simulink model "ACC"  (Simulink 7.4)
settings: Solver=ode45  StartTime=0.0  StopTime=100  RelTol=1e-3
values from neighbouring files (symbols this model uses):
  A = ACC_cont.A    [pritam_acc.m]
  ACCController_name = 'ACCController'    [pritam_acc.m]
  B = ACC_cont.B    [pritam_acc.m]
  Bd = ACC_cont.C    [pritam_acc.m]
  uini = 0    [pritam_acc.m]
  xini = [40;29;30]    [pritam_acc.m]
libraries: simulink x1
settings Model: Creator=manuelmazo  LastModifiedBy=p261584  ExtModeAutoUpdateStatusClock=off
settings OptimizationCC: InitFltsAndDblsToZero=on
settings DebuggingCC: SaveWithParameterizedLinksMsg=none
settings GRTTargetCC: TargetFcnLib=ansi_tfl_tmw.mat

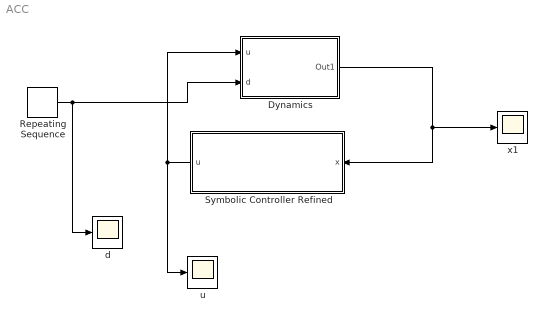
== system ACC ==
  Dynamics : Subsystem
  Repeating Sequence : simulink/Sources/Repeating Sequence  SystemSampleTime=-1  rep_seq_t=[0 0.2]  rep_seq_y=[-0.1 -0.1]
  Symbolic Controller Refined : Subsystem  mask{contr_name=ACCController_name, uini=uini}
      mask prompts: contr_name "Controller Name"; uini "Initial Controller State"
      mask init:
      | load(strcat(contr_name,'_symb'), 'params_symb');
  d : Scope
      settings: YMin=-0.1  YMax=-0.1
  u : Scope
      settings: YMin=-1  YMax=1  SaveName=ScopeData3
  x1 : Scope
      settings: YMin=25  YMax=65
  wires:
  Dynamics/1(Out1) -> Symbolic Controller Refined/1(x), x1/1
  Symbolic Controller Refined/1(u) -> u/1, Dynamics/1(u)
  Repeating Sequence/1 -> Dynamics/2(d), d/1

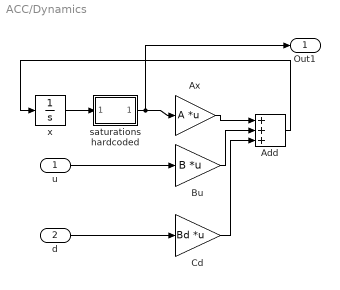
== system ACC/Dynamics ==
  u : Inport  OutDataType=sfix(16)  OutScaling=2^0
  d : Inport  Port=2  OutDataType=sfix(16)  OutScaling=2^0
  Add : Sum  Inputs=+++  OutDataType=sfix(16)  OutScaling=2^-10
  Ax : Gain  Gain=A  Multiplication=Matrix(K*u) (u vector)  ParameterDataType=sfix(16)  ParameterScaling=2^0  OutDataType=sfix(16)  OutScaling=2^0
  Bu : Gain  Gain=B  Multiplication=Matrix(K*u)  ParameterDataType=sfix(16)  ParameterScaling=2^0  OutDataType=sfix(16)  OutScaling=2^0
  Cd : Gain  Gain=Bd  Multiplication=Matrix(K*u)  ParameterDataType=sfix(16)  ParameterScaling=2^0  OutDataType=sfix(16)  OutScaling=2^0
  saturations hardcoded : Subsystem
  x : Integrator  InitialCondition=xini
  Out1 : Outport  OutDataType=sfix(16)  OutScaling=2^0
  wires:
  x/1 -> saturations hardcoded/1(In1)
  Ax/1 -> Add/1
  Bu/1 -> Add/2
  Add/1 -> x/1
  u/1 -> Bu/1
  saturations hardcoded/1(Out1) -> Ax/1, Out1/1
  d/1 -> Cd/1
  Cd/1 -> Add/3

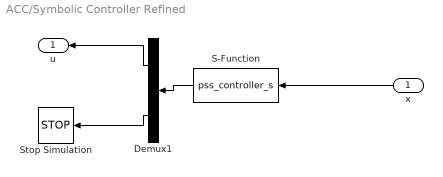
== system ACC/Symbolic Controller Refined ==
  x : Inport  OutDataType=sfix(16)  OutScaling=2^0
  Demux1 : Demux  Outputs=2
  S-Function : S-Function  FunctionName=pss_controller_s  Parameters=params_symb, contr_name, uini  EnableBusSupport=off
  Stop Simulation : Stop
  u : Outport  OutDataType=sfix(16)  OutScaling=2^0
  wires:
  S-Function/1 -> Demux1/1
  x/1 -> S-Function/1
  Demux1/1 -> u/1
  Demux1/2 -> Stop Simulation/1

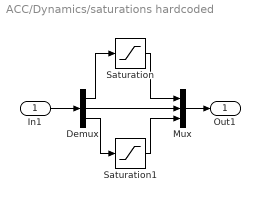
== system ACC/Dynamics/saturations hardcoded ==
  In1 : Inport  OutDataType=sfix(16)  OutScaling=2^0
  Demux : Demux  Outputs=3
  Mux : Mux  Inputs=3
  Saturation : Saturate  UpperLimit=70  LowerLimit=0
  Saturation1 : Saturate  UpperLimit=30  LowerLimit=28
  Out1 : Outport  OutDataType=sfix(16)  OutScaling=2^0
  wires:
  In1/1 -> Demux/1
  Demux/1 -> Saturation/1
  Demux/3 -> Saturation1/1
  Saturation1/1 -> Mux/3
  Saturation/1 -> Mux/1
  Demux/2 -> Mux/2
  Mux/1 -> Out1/1
